simulink model "gmsk_tx"  (Simulink 7.9)
settings: Solver=FixedStepDiscrete  SolverMode=SingleTasking  StartTime=0.0  StopTime=1e2  RelTol=1e-3
model workspace (MAT data in the model file):
  Sig = Simulink.Signal
  Sig.DataType = 'auto'
  Sig.Dimensions = -1
  Sig.DimensionsMode = 'auto'
  Sig.Complexity = 'auto'
  Sig.SampleTime = -1
  Sig.SamplingMode = 'auto'
  sin_lut_length = Simulink.Parameter
  sin_lut_length.Value = 64
  sin_lut_length.DataType = 'auto'
  Sig1 = Simulink.Signal
  Sig1.DataType = 'auto'
  Sig1.Dimensions = -1
  Sig1.DimensionsMode = 'auto'
  Sig1.Complexity = 'auto'
  Sig1.SampleTime = -1
  Sig1.SamplingMode = 'auto'
PreLoadFcn:
  | gmsk_syn_init;
undefined symbols (not defined in the file or in its folder): gaussfir, gmsk_syn_params
libraries: shlslibv1 x13
settings Model: synDspstartup=OK  Creator=sszilvasi  LastModifiedBy=sszilvasi
settings DataIOCC: SaveOutput=off  SignalLogging=off  SaveTime=off
settings OptimizationCC: InlineParams=on
settings DebuggingCC: AlgebraicLoopMsg=error  InheritedTsInSrcMsg=none

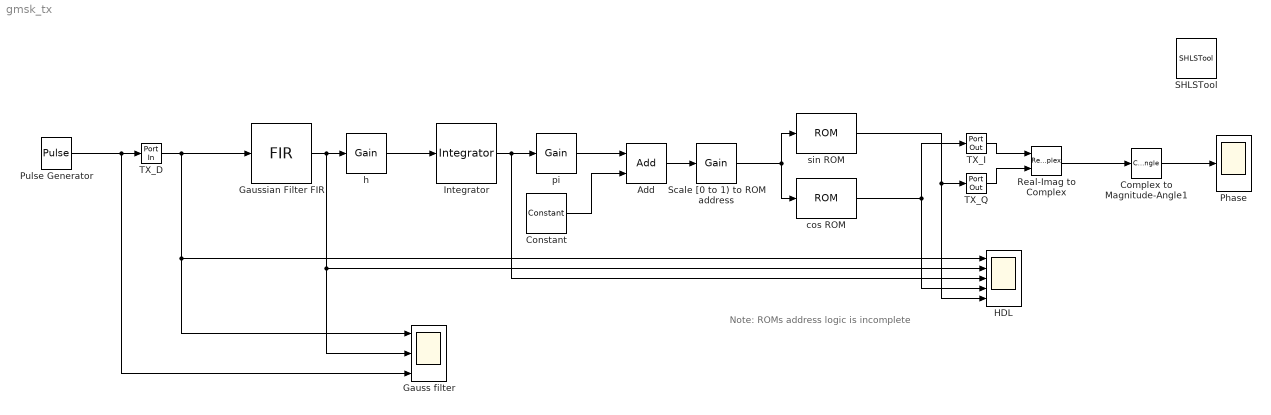
== system gmsk_tx ==
  note: Note: ROMs address logic is incomplete
  Add : shlslibv1/Math Functions/Add  syn_add_opr=++  syn_out_f=Automatic  syn_out_wl=5  syn_out_fl=5  syn_out_dt=unsigned  syn_out_sat=off  syn_out_rnd=Floor (Truncate)  synBlockType=primitive  synLatency=0  synBlockId=96  syn_sum_of_rows=off
  Complex to Magnitude-Angle1 : ComplexToMagnitudeAngle  Output=Angle
  Constant : shlslibv1/Sources/Constant  syn_cst_val=.5  syn_cst_fl=1  syn_cst_dt=signed  syn_cst_rnd=on  syn_cst_st=-1  synBlockType=primitive  synLatency=0  synBlockId=15
  Gauss filter : Scope  NumInputPorts=3
      settings: YMin=-5~-5~-5  YMax=5~5~5
  Gaussian Filter FIR : shlslibv1/Filtering/FIR  syn_coef_vec=gaussfir(0.5,1,8)  syn_coef_fl=15  syn_coef_rnd=Nearest  syn_show_q=off  syn_dp_f=Automatic  syn_dp_wl=16  syn_dp_fl=8  syn_dp_sat=off  syn_dp_rnd=Floor (Truncate)  syn_out_f=Full Precision  syn_out_wl=16  syn_out_fl=8  syn_out_dt=signed  syn_out_sat=off  syn_out_rnd=Floor (Truncate)  syn_rst_port=off  syn_en_port=off  synBlockType=primitive  synLatency=0  synBlockId=80
  HDL : Scope  NumInputPorts=5
      settings: YMin=-5~-5~-5~-5~-5  YMax=5~5~5~5~5
  Integrator : shlslibv1/Filtering/Integrator  syn_pole_val=1  syn_feedback_fl=8  syn_out_f=Automatic  syn_out_wl=16  syn_out_fl=8  syn_out_dt=signed  syn_out_sat=off  syn_out_rnd=off  syn_rst_port=off  syn_en_port=off  synBlockType=custom  synLatency=0
  Phase : Scope
      settings: SaveName=ScopeData5
  Pulse Generator : DiscretePulseGenerator  Amplitude=-1  Period=100  PhaseDelay=10
  Real-Imag to Complex : RealImagToComplex
  SHLSTool : shlslibv1/SHLSTool  synBlockType=tool  syn_dsp_mode=FPGA
  Scale [0 to 1) to ROM address : shlslibv1/Math Functions/Gain  syn_gain_val=sin_lut_length  syn_gain_fl=15  syn_gain_dt=signed  syn_gain_rnd=on  syn_out_f=Specify  syn_out_wl=6  syn_out_fl=0  syn_out_dt=unsigned  syn_out_sat=off  syn_out_rnd=Floor (Truncate)  synBlockType=primitive  synLatency=0  synBlockId=3  syn_opr_mode=0
  TX_D : shlslibv1/Ports & Subsystems/Port In  syn_out_wl=16  syn_out_fl=14  syn_out_dt=signed  syn_out_st=1/30e6  syn_capture=on  syn_register=off  syn_out_sat=off  syn_out_rnd=on  synBlockType=port  synLatency=0  synBlockId=0
  TX_I : shlslibv1/Ports & Subsystems/Port Out  syn_capture=on  syn_register=off  synBlockType=port  synLatency=0  synBlockId=1
  TX_Q : shlslibv1/Ports & Subsystems/Port Out  syn_capture=on  syn_register=off  synBlockType=port  synLatency=0  synBlockId=1
  cos ROM : shlslibv1/Memories/ROM  syn_rom_vec=cos(pi*2*[0:sin_lut_length-1]/sin_lut_length)  syn_out_wl=10  syn_out_fl=8  syn_out_dt=signed  syn_out_sat=on  syn_out_rnd=on  synBlockType=primitive  synLatency=1  synBlockId=62
  h : shlslibv1/Math Functions/Gain  syn_gain_val=1/4  syn_gain_fl=15  syn_gain_dt=signed  syn_gain_rnd=on  syn_out_f=Full Precision  syn_out_wl=16  syn_out_fl=8  syn_out_dt=signed  syn_out_sat=off  syn_out_rnd=Floor (Truncate)  synBlockType=primitive  synLatency=0  synBlockId=3  syn_opr_mode=0
  pi : shlslibv1/Math Functions/Gain  syn_gain_val=1/gmsk_syn_params.N  syn_gain_fl=15  syn_gain_dt=signed  syn_gain_rnd=on  syn_out_f=Full Precision  syn_out_wl=16  syn_out_fl=8  syn_out_dt=signed  syn_out_sat=off  syn_out_rnd=Floor (Truncate)  synBlockType=primitive  synLatency=0  synBlockId=3  syn_opr_mode=0
  sin ROM : shlslibv1/Memories/ROM  syn_rom_vec=sin(pi*2*[0:gmsk_syn_params.sin_lut_length-1]/gmsk_syn_params.sin_lut_length)  syn_out_wl=10  syn_out_fl=8  syn_out_dt=signed  syn_out_sat=on  syn_out_rnd=on  synBlockType=primitive  synLatency=1  synBlockId=62
  wires:
  Gaussian Filter FIR/1 -> h/1, HDL/2, Gauss filter/2
  TX_I/1 -> Real-Imag to Complex/1
  TX_Q/1 -> Real-Imag to Complex/2
  h/1 -> Integrator/1
  Integrator/1 -> pi/1, HDL/3
  Add/1 -> Scale [0 to 1) to ROM address/1
  cos ROM/1 -> TX_I/1, HDL/4
  sin ROM/1 -> HDL/5, TX_Q/1
  Real-Imag to Complex/1 -> Complex to Magnitude-Angle1/1
  pi/1 -> Add/1
  Constant/1 -> Add/2
  Scale [0 to 1) to ROM address/1 -> sin ROM/1, cos ROM/1
  TX_D/1 -> HDL/1, Gauss filter/1, Gaussian Filter FIR/1
  Pulse Generator/1 -> TX_D/1, Gauss filter/3
  Complex to Magnitude-Angle1/1 -> Phase/1
